simulink model "parte3_eje4_avr_exac1v2013"  (Simulink 8.1)
settings: Solver=ode45  SolverMode=SingleTasking  StartTime=0.0  StopTime=10  RelTol=1e-3
values from neighbouring files (symbols this model uses):
  AEX = 0.014    [parte3_DC1A_data.m]    (also in parte3_eje3_EXAC1.m = 0.1; parte3_eje3_EXAC2.m = 0.1)
  BEX = 1.55    [parte3_DC1A_data.m]    (also in parte3_eje3_EXAC1.m = 0.03; parte3_eje3_EXAC2.m = 0.03)
  IFDfin = 1000    [parte3_eje3_EXAC1.m]    (also in parte3_eje3_EXAC2.m = 0; parte3_eje5_ESSTB.m = 1)
  Ka = 400    [parte3_eje3_EXAC1.m]    (also in parte3_eje3_EXAC2.m)
  KC = 0.2    [parte3_eje3_EXAC1.m]    (also in parte3_eje3_EXAC2.m; parte3_eje5_ESSTB.m = 0.1; parte3_eje6_ESST1A.m = 0.01)
  KD = 0.38    [parte3_eje3_EXAC1.m]    (also in parte3_eje3_EXAC2.m)
  Ke = 1    [parte3_eje3_EXAC1.m]    (also in parte3_eje3_EXAC2.m)
  Kf = 0.03    [parte3_eje3_EXAC1.m]    (also in parte3_eje3_EXAC2.m)
  Ta = 0.02    [parte3_eje3_EXAC1.m]    (also in parte3_eje3_EXAC2.m; parte3_eje5_ESSTB.m = 0.01)
  Tb = 2    [parte3_eje3_EXAC1.m]    (also in parte3_eje3_EXAC2.m)
  Tc = 2    [parte3_eje3_EXAC1.m]    (also in parte3_eje3_EXAC2.m)
  Te = 0.8    [parte3_eje3_EXAC1.m]    (also in parte3_eje3_EXAC2.m)
  Tf = 1    [parte3_eje3_EXAC1.m]    (also in parte3_eje3_EXAC2.m)
  Tr = 0.01    [parte3_eje2_SMIB_Exc_graph.m]    (also in parte3_eje3_EXAC1.m; parte3_eje3_EXAC2.m; parte3_eje5_ESSTB.m = 0.3)
  Vrefin = 1    [parte3_eje3_EXAC1.m]    (also in parte3_eje3_EXAC2.m; parte3_eje5_ESSTB.m = 0.01)
  Vrmax = 15    [parte3_eje3_EXAC1.m]    (also in parte3_eje3_EXAC2.m)
  Vrmin = -15    [parte3_eje3_EXAC1.m]    (also in parte3_eje3_EXAC2.m)
settings Model: Creator=cjuar  LastModifiedBy=cjuar  CovMetricSettings=dwe  CovHtmlReporting=off  covSaveCumulativeToWorkspaceVar=off  CovSaveSingleToWorkspaceVar=off  CovExternalEMLEnable=on
settings DataIOCC: LimitDataPoints=off  SaveFormat=StructureWithTime  SignalLoggingSaveFormat=Dataset
settings OptimizationCC: ExpressionDepthLimit=128
settings DebuggingCC: UnderspecifiedInitializationDetection=Simplified  MergeDetectMultiDrivingBlocksExec=error  SolverPrmCheckMsg=none  FcnCallInpInsideContextMsg=EnableAllAsError  FrameProcessingCompatibilityMsg=error  StateNameClashWarn=none  SFUnexpectedBacktrackingDiag=error  SFNoUnconditionalDefaultTransitionDiag=error
settings HardwareCC: ProdBitPerPointer=64  ProdLargestAtomicFloat=Float  ProdIntDivRoundTo=Zero  ProdEndianess=LittleEndian  ProdHWDeviceType=Specified
settings ModelReferenceCC: PropagateSignalLabelsOutOfModel=on
settings GRTTargetCC: CodeReplacementLibrary=C99 (ISO)  GeneratePreprocessorConditionals=Use local settings  CombineOutputUpdateFcns=on  GRTInterface=off

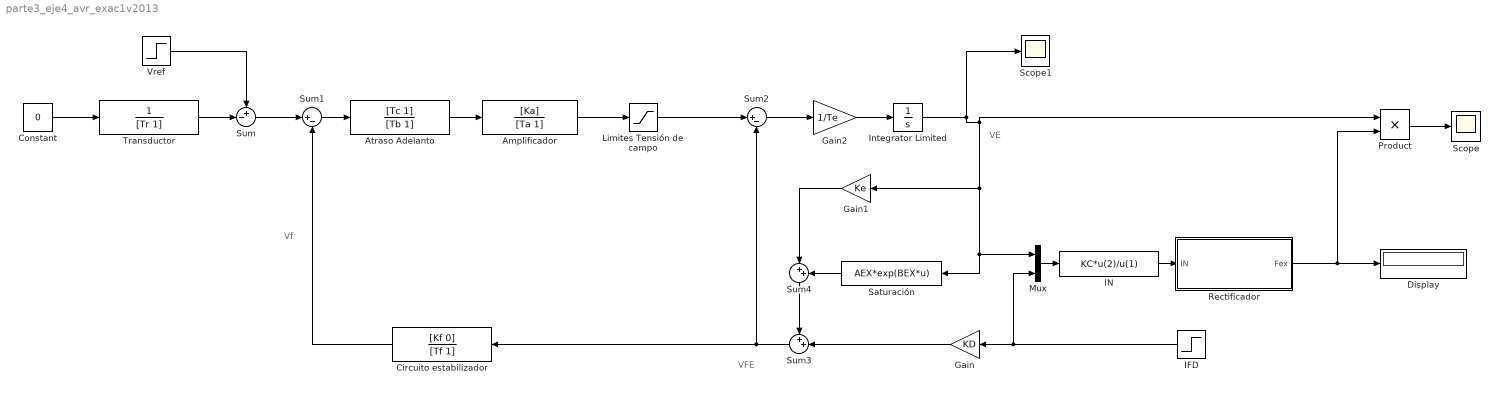
== system parte3_eje4_avr_exac1v2013 ==
  note: VE
  note: VFE
  note: Vf
  Amplificador : TransferFcn  Numerator=[Ka]  Denominator=[Ta 1]
  Atraso Adelanto : TransferFcn  Numerator=[Tc 1]  Denominator=[Tb 1]
  Circuito estabilizador : TransferFcn  Numerator=[Kf 0]  Denominator=[Tf 1]
  Constant : Constant  Value=0
  Display : Display
  Gain : Gain  Gain=KD
  Gain1 : Gain  Gain=Ke
  Gain2 : Gain  Gain=1/Te
  IFD : Step  After=IFDfin  SampleTime=0
  IN : Fcn  Expr=KC*u(2)/u(1)
  Integrator Limited : Integrator  LimitOutput=on  UpperSaturationLimit=100  LowerSaturationLimit=0
  Limites Tensión de campo : Saturate  UpperLimit=Vrmax  LowerLimit=Vrmin
  Mux : Mux  Inputs=2
  Product : Product
  Rectificador : MATLAB Function  TreatAsAtomicUnit=on
      settings: PermitHierarchicalResolution=ParametersOnly
  Saturación : Fcn  Expr=AEX*exp(BEX*u)
  Scope : Scope
      settings: TimeRange=auto  MaxDataPoints=5000  SaveToWorkspace=off  SaveName=ScopeData  YMin=-1.00000  YMax=1.00000  SampleTime=-1
  Scope1 : Scope
      settings: TimeRange=auto  MaxDataPoints=5000  SaveToWorkspace=off  YMin=-1.38256  YMax=12.44308  SampleTime=-1
  Sum : Sum  Inputs=+-|
  Sum1 : Sum  Inputs=|+-
  Sum2 : Sum  Inputs=|+-
  Sum3 : Sum  Inputs=++|
  Sum4 : Sum  Inputs=|++
  Transductor : TransferFcn  Denominator=[Tr 1]
  Vref : Step  After=Vrefin  SampleTime=0
  wires:
  Amplificador/1 -> Limites Tensión de campo/1
  Atraso Adelanto/1 -> Amplificador/1
  Circuito estabilizador/1 -> Sum1/2
  Sum/1 -> Sum1/1
  Transductor/1 -> Sum/2
  Constant/1 -> Transductor/1
  Vref/1 -> Sum/1
  Sum1/1 -> Atraso Adelanto/1
  Limites Tensión de campo/1 -> Sum2/1
  Gain/1 -> Sum3/2
  Gain1/1 -> Sum4/1
  Saturación/1 -> Sum4/2
  Sum2/1 -> Gain2/1
  Integrator Limited/1 -> Product/1, Mux/1, Saturación/1, Gain1/1, Scope1/1
  IFD/1 -> Mux/2, Gain/1
  Mux/1 -> IN/1
  IN/1 -> Rectificador/1(IN)
  Rectificador/1(Fex) -> Product/2, Display/1
  Sum4/1 -> Sum3/1
  Sum3/1 -> Sum2/2, Circuito estabilizador/1
  Product/1 -> Scope/1
  Gain2/1 -> Integrator Limited/1

== matlab function Rectificador ==
  data: IN input double; Fex output double
function Fex = Rectificador(IN)
if IN<=0
    Fex=1;
elseif IN<=0.433
    Fex=1-0.577*IN;
elseif IN>0.433&&IN<0.75
    Fex=sqrt(0.75-IN^2);
elseif IN>=0.75&&IN<=1
    Fex=1.732*(1-IN);
else
    Fex=0;
end
